simulink model "P4_RaspberryModel_with_DT"  (R2025b)
settings: Solver=daessc  StartTime=0.0  StopTime=Inf  FixedStep=0.01  RelTol=1e-3
PreLoadFcn:
  | % Kalman Filter testing
  | m=0.370;
  | l=0.075; %0.079793%determined by pendulum experiment %former values 0.032, 0.035;
  | lm=l*m; %lm=0.032*0.377
  | r=0.0405;
  | rm=r*m; %rm=0.0405*0.377
  | K=1;
  | 
  | tem=0.2 %initial guess
  | eta=2*lm+rm+(2*m*l^2/r);
  | 
  | A31=(lm+rm)/(tem*eta);
  | A32=9.81*lm/(r*eta);
  | A=[0 1 0 0; 0 -1/tem, 0, 0; 0, 0, 0, 1; 0 A31, A32, 0];
  | B=[0; 1/tem;0;-A31];
model workspace (MAT data in the model file):
  Amp = 1
undefined symbols (not defined in the file): anglerate, DiscIntNeverNeededParam, motor_left, motor_param, motor_right, PosEnc, VelEnc
libraries: simulink x19, raspberrypiCommlib x7, dspstat3 x6, slpidlib x3, sm_lib x3, raspberrypiNetworklib x2, svdutilitieslib x2, SigiLib x2, robotcorelib x1, mspfiltlib x1, nesl_utility x1
(part 2 of 2)

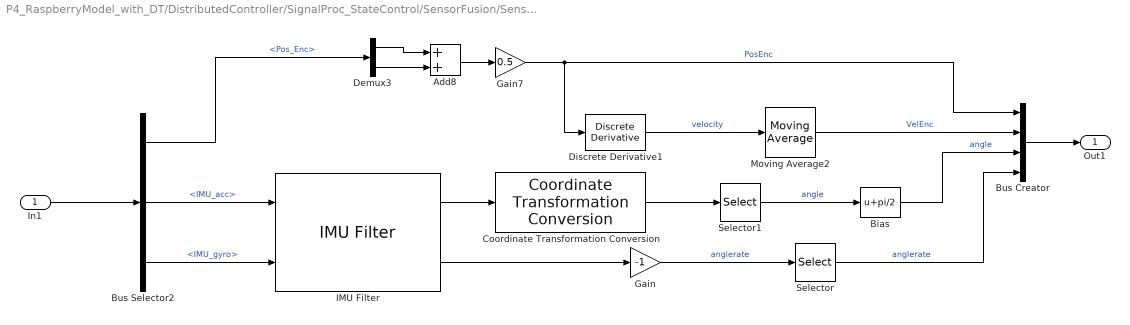
== system P4_RaspberryModel_with_DT/DistributedController/SignalProc_StateControl/SensorFusion/SensorFusion ==
  In1 : Inport
  Add8 : Sum
  Bias : Bias  Bias=pi/2  SaturateOnIntegerOverflow=off
  Bus Creator : BusCreator  Inputs=PosEnc,VelEnc,angle,anglerate  OutDataTypeStr=Bus: States
  Bus Selector2 : BusSelector  OutputSignals=Pos_Enc,IMU_acc,IMU_gyro
  Coordinate Transformation Conversion : robotcorelib/Coordinate Transformation Conversion  InputRepresentation=Rotation Matrix  InputEulerSequence=ZYX  ShowTrVecInputPort=on  OutputRepresentation=Euler Angles  OutputEulerSequence=XYZ  ShowTrVecOutputPort=on  SimulateUsing=Interpreted execution
      settings: LibrarySourceBlock=navlib/Utilities/Coordinate Transformation Conversion
  Demux3 : Demux  Outputs=2
  Discrete Derivative1 : simulink/Discrete/Discrete Derivative  gainval=1.0  ICPrevScaledInput=0.0  OutMin=[]  OutMax=[]  OutDataType=fixdt(1, 16)  OutScaling=2^-10  DoSatur=off
  Gain : Gain  Gain=-1
  Gain7 : Gain  Gain=0.5
  IMU Filter : mspfiltlib/IMU Filter  DispRefFrame=NED  OrientationFormat=Rotation matrix  DecimationFactor=1  InitialProcessNoise=imufilter.defaultProcessNoise  AccelerometerNoise=2.2693e-4  GyroscopeNoise=2.4065e-5  GyroscopeDriftNoise=3.0462e-13  LinearAccelerationNoise=0.0096236100000000012  LinearAccelerationDecayFactor=0.5  SimulateUsing=Interpreted execution
  Moving Average2 : dspstat3/Moving Average  Method=Sliding window  ForgettingFactorPort=off  SpecifyWindowLength=on  WindowLength=4  OverlapLength=3  AllowArbitraryInputLength=off  ForgettingFactor=0.9  SimulateUsing=Interpreted execution
  Selector : Selector  InputPortWidth=3  IndexOptions=Index vector (dialog)  Indices=[1]  OutputSizes=1
  Selector1 : Selector  InputPortWidth=3  IndexOptions=Index vector (dialog)  Indices=[1]  OutputSizes=1
  Out1 : Outport  OutDataTypeStr=Bus: States
  wires:
  Gain7/1 -> Bus Creator/1, Discrete Derivative1/1  "PosEnc"
  Demux3/2 -> Add8/2
  Discrete Derivative1/1 -> Moving Average2/1  "velocity"
  Bus Selector2/1 -> Demux3/1  "<Pos_Enc>"
  IMU Filter/1 -> Coordinate Transformation Conversion/1
  IMU Filter/2 -> Gain/1
  Bus Selector2/2 -> IMU Filter/1  "<IMU_acc>"
  Add8/1 -> Gain7/1
  Selector1/1 -> Bias/1  "angle"
  Bus Selector2/3 -> IMU Filter/2  "<IMU_gyro>"
  Demux3/1 -> Add8/1
  Coordinate Transformation Conversion/1 -> Selector1/1
  Selector/1 -> Bus Creator/4  "anglerate"
  Bus Creator/1 -> Out1/1
  In1/1 -> Bus Selector2/1
  Moving Average2/1 -> Bus Creator/2  "VelEnc"
  Bias/1 -> Bus Creator/3  "angle"
  Gain/1 -> Selector/1  "anglerate"

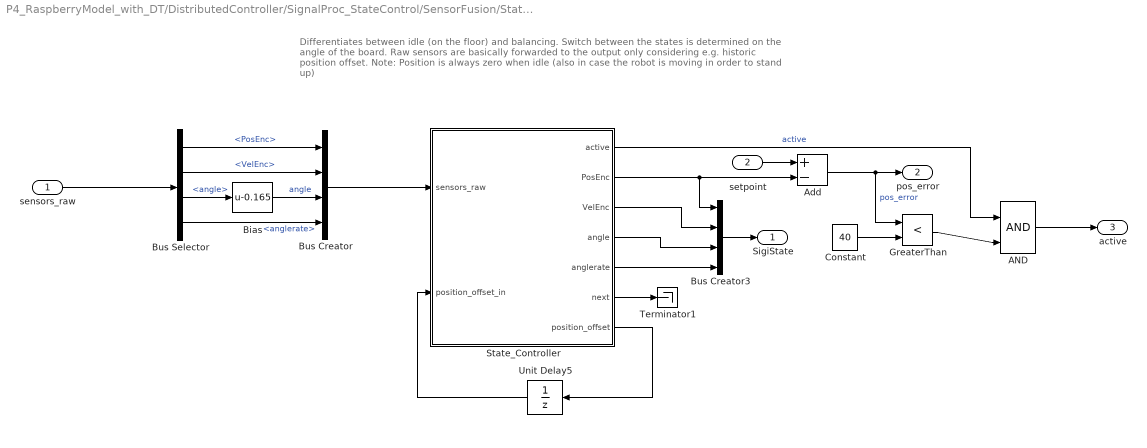
== system P4_RaspberryModel_with_DT/DistributedController/SignalProc_StateControl/SensorFusion/Statemachine ==
  note: Differentiates between idle (on the floor) and balancing.
      | Switch between the states is determined on the angle of the board.
      | Raw sensors are basically forwarded to the output only considering e.g. historic position offset.
      | Note: Position is always zero when idle (also in case the robot is moving in order to stand up)
  sensors_raw : Inport
  setpoint : Inport  Port=2
  AND : Logic  IconShape=distinctive  AllPortsSameDT=off  OutDataTypeStr=boolean
  Add : Sum  Inputs=+-
  Bias : Bias  Bias=-0.165  SaturateOnIntegerOverflow=off
  Bus Creator : BusCreator  Inputs=4  OutDataTypeStr=Bus: States
  Bus Creator3 : BusCreator  Inputs=PosEnc,VelEnc,angle,anglerate  OutDataTypeStr=Bus: States
  Bus Selector : BusSelector  OutputSignals=PosEnc,VelEnc,angle,anglerate
  Constant : Constant  Value=40  SampleTime=0.01
  GreaterThan : RelationalOperator  Operator=<  OutDataTypeStr=boolean  RndMeth=Simplest  InputSameDT=off
  State_Controller : Stateflow chart  TreatAsAtomicUnit=on
      settings: PortSchema="{\"entries\":[{\"content\":{\"sides\":[{\"content\":{\"connectorIds\":[\"In1\",\"In2\"]},\"type\":\"ConnectorPlacement.EquallySpacedRectSide\",\"uuid\":\"eb7aab9b-7b76-4287-a386-1fa94ac59388\"},{\"content\":{\"connectorIds\":[\"Out1\",\"Out4\",\"Out6\",\"Out5\",\"Out7\",\"Out2\",\"Out3\"],\"side\":\"RIGHT\"},\"type\":\"ConnectorPlacement.EquallySpacedRectSide\",\"uuid\":\"6af62896-360c-441a-abcb-d94064922169\"},{\"content\":{\"side\":\"TOP\"},\"type\":\"ConnectorPlacement.EquallySpacedRectSide\",\"uuid\":\"2e15ba59-a93a-45bf-98f2-d7da7205ed1e\"}]},\"type\":\"ConnectorPlacement.EquallySpacedConnector\",\"uuid\":\"1bfad314-89c0-4ae7-b541-c4839d2ff64d\"}],\"packageUris\":[\"http://schema.mathworks.com/mf0/Connector/R2020b\"],\"version\":\"1.0\"}"
  Terminator1 : Terminator
  Unit Delay5 : UnitDelay  SampleTime=-1  HasFrameUpgradeWarning=on
  SigiState : Outport  OutDataTypeStr=Bus: States
  pos_error : Outport  Port=2
  active : Outport  Port=3
  wires:
  Unit Delay5/1 -> State_Controller/2(position_offset_in)
  Bus Creator3/1 -> SigiState/1
  State_Controller/7(anglerate) -> Bus Creator3/4
  State_Controller/3(position_offset) -> Unit Delay5/1
  State_Controller/5(angle) -> Bus Creator3/3
  sensors_raw/1 -> Bus Selector/1
  State_Controller/4(PosEnc) -> Bus Creator3/1, Add/2
  State_Controller/1(active) -> AND/1  "active"
  State_Controller/2(next) -> Terminator1/1
  setpoint/1 -> Add/1
  Add/1 -> GreaterThan/1, pos_error/1  "pos_error"
  Constant/1 -> GreaterThan/2
  GreaterThan/1 -> AND/2
  AND/1 -> active/1
  State_Controller/6(VelEnc) -> Bus Creator3/2
  Bus Selector/3 -> Bias/1  "<angle>"
  Bias/1 -> Bus Creator/3  "angle"
  Bus Selector/4 -> Bus Creator/4  "<anglerate>"
  Bus Selector/2 -> Bus Creator/2  "<VelEnc>"
  Bus Selector/1 -> Bus Creator/1  "<PosEnc>"
  Bus Creator/1 -> State_Controller/1(sensors_raw)

== system P4_RaspberryModel_with_DT/SegwayDigitalTwin/RaspberryImplementation/LSM6DS33_IMU/Initialize Function ==
  note: Initiate the IMU - Setting sample rate and sensor range
  Constant : Constant  Value=64
  Constant2 : Constant  Value=64
  Data Type Conversion : DataTypeConversion  OutDataTypeStr=uint8  SaturateOnIntegerOverflow=off  RndMeth=Floor
  Data Type Conversion1 : DataTypeConversion  OutDataTypeStr=uint8  SaturateOnIntegerOverflow=off  RndMeth=Floor
  Event Listener : EventListener  DisableCoverage=on  EventName=reset
  I2C acc write : raspberrypiCommlib/I2C Controller Write  BoardProperty=Pi 3 Model B+  I2CModule=1  Mode=Master  SlaveAddress=107  SlaveByteOrder=BigEndian  Direction=Transmitter  RegisterAddressMode=on  RegisterAddress=16  SlaveDataType=uint8  DataLength=1  NoAck=off  RepeatedStart=off  OutputStatus=off
  I2C gyro write : raspberrypiCommlib/I2C Controller Write  BoardProperty=Pi 3 Model B+  I2CModule=1  Mode=Master  SlaveAddress=107  SlaveByteOrder=BigEndian  Direction=Transmitter  RegisterAddressMode=on  RegisterAddress=17  SlaveDataType=uint8  DataLength=1  NoAck=off  RepeatedStart=off  OutputStatus=off
  wires:
  Constant2/1 -> Data Type Conversion/1
  Data Type Conversion/1 -> I2C gyro write/1
  Data Type Conversion1/1 -> I2C acc write/1
  Constant/1 -> Data Type Conversion1/1

== system P4_RaspberryModel_with_DT/SegwayDigitalTwin/RaspberryImplementation/LSM6DS33_IMU/Terminate Function ==
  Constant : Constant  Value=0
  Constant2 : Constant  Value=0
  Data Type Conversion1 : DataTypeConversion  OutDataTypeStr=uint8  SaturateOnIntegerOverflow=off  RndMeth=Floor
  Data Type Conversion2 : DataTypeConversion  OutDataTypeStr=uint8  SaturateOnIntegerOverflow=off  RndMeth=Floor
  Event Listener : EventListener  DisableCoverage=on  EventType=Terminate  EventName=reset
  I2C Master Write : raspberrypiCommlib/I2C Controller Write  BoardProperty=Pi 3 Model B+  I2CModule=1  Mode=Master  SlaveAddress=107  SlaveByteOrder=BigEndian  Direction=Transmitter  RegisterAddressMode=on  RegisterAddress=17  SlaveDataType=uint8  DataLength=1  NoAck=off  RepeatedStart=off  OutputStatus=off
  I2C Master Write2 : raspberrypiCommlib/I2C Controller Write  BoardProperty=Pi 3 Model B+  I2CModule=1  Mode=Master  SlaveAddress=107  SlaveByteOrder=BigEndian  Direction=Transmitter  RegisterAddressMode=on  RegisterAddress=16  SlaveDataType=uint8  DataLength=1  NoAck=off  RepeatedStart=off  OutputStatus=off
  wires:
  Data Type Conversion1/1 -> I2C Master Write/1
  Constant/1 -> Data Type Conversion2/1
  Data Type Conversion2/1 -> I2C Master Write2/1
  Constant2/1 -> Data Type Conversion1/1

== system P4_RaspberryModel_with_DT/DistributedController/SignalProc_StateControl/ClassicalCalibration/SensorProcessing/BoardAngle ==
  note: This model only calculates the angle by comparing the relative magnitude of each component.
      | For the absolute acceleration one would need to use a calibration gain of 0.000488. (but sensor might drift...)
  x-sens : Inport  OutDataTypeStr=double
  z-sens : Inport  Port=2  OutDataTypeStr=double
  Atan2 : Trigonometry  Operator=atan2
  Gain1 : Gain  Commented=through  Gain=0.000488
  Gain2 : Gain  Commented=through  Gain=0.000488
  low pass filter : simulink/Discrete/Transfer Fcn First Order  PoleZ=0.95  ICPrevOutput=0.0  DoSatur=off
  Outport : Outport
  wires:
  x-sens/1 -> Gain2/1
  Gain1/1 -> Atan2/1
  Gain2/1 -> Atan2/2
  z-sens/1 -> Gain1/1
  Atan2/1 -> low pass filter/1  "board angle [rad]"
  low pass filter/1 -> Outport/1

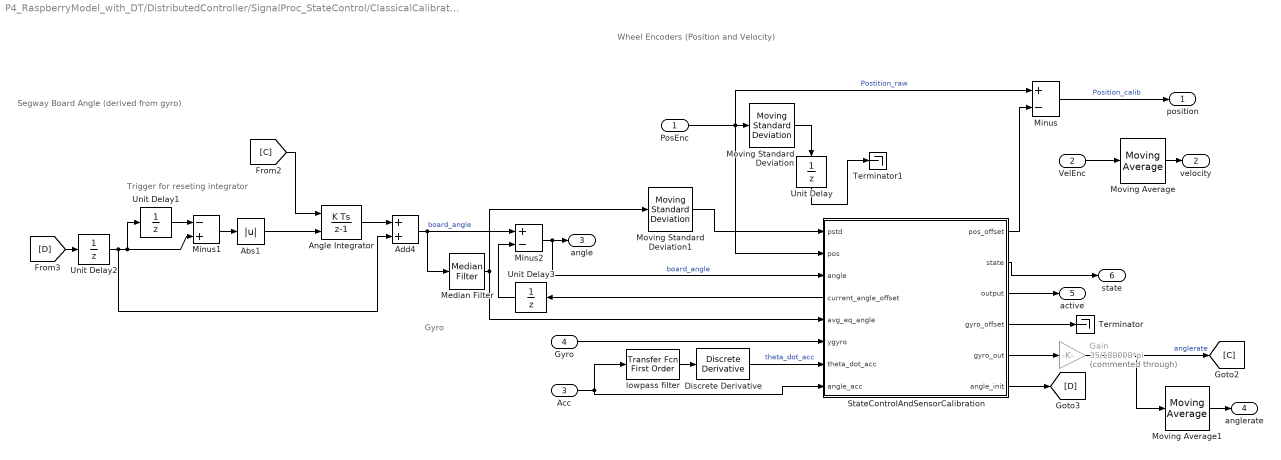
== system P4_RaspberryModel_with_DT/DistributedController/SignalProc_StateControl/ClassicalCalibration/Statemachine_Old/StateControl ==
  note: Segway Board Angle (derived from gyro)
  note: Wheel Encoders (Position and Velocity)
  note: Gyro
  note: Trigger for reseting integrator
  PosEnc : Inport
  VelEnc : Inport  Port=2
  Acc : Inport  Port=3
  Gyro : Inport  Port=4
  Abs1 : Abs  SaturateOnIntegerOverflow=off
  Add4 : Sum
  Angle Integrator : DiscreteIntegrator  gainval=1  ExternalReset=either  SampleTime=-1  ICPrevOutput=DiscIntNeverNeededParam  ICPrevScaledInput=DiscIntNeverNeededParam
  Discrete Derivative : simulink/Discrete/Discrete Derivative  gainval=1  ICPrevScaledInput=0.0  OutMin=[]  OutMax=[]  OutDataType=fixdt(1, 16)  OutScaling=2^-10  DoSatur=off
  Gain : Gain  Commented=through  Gain=35/180000*pi
  Median Filter : dspstat3/Median Filter  WindowLength=200  SimulateUsing=Interpreted execution
  Minus : Sum  Inputs=+-
  Minus1 : Sum  Inputs=-+
  Minus2 : Sum  Inputs=+-
  Moving Average : dspstat3/Moving Average  Method=Sliding window  ForgettingFactorPort=off  SpecifyWindowLength=on  WindowLength=4  OverlapLength=3  AllowArbitraryInputLength=off  ForgettingFactor=0.9  SimulateUsing=Code generation
  Moving Average1 : dspstat3/Moving Average  Method=Sliding window  ForgettingFactorPort=off  SpecifyWindowLength=on  WindowLength=4  OverlapLength=3  AllowArbitraryInputLength=off  ForgettingFactor=0.9  SimulateUsing=Code generation
  Moving Standard Deviation : dspstat3/Moving Standard Deviation  Method=Sliding window  ForgettingFactorPort=off  SpecifyWindowLength=on  WindowLength=200  OverlapLength=199  AllowArbitraryInputLength=off  ForgettingFactor=0.9  SimulateUsing=Code generation
  Moving Standard Deviation1 : dspstat3/Moving Standard Deviation  Method=Sliding window  ForgettingFactorPort=off  SpecifyWindowLength=on  WindowLength=200  OverlapLength=199  AllowArbitraryInputLength=off  ForgettingFactor=0.9  SimulateUsing=Code generation
  StateControlAndSensorCalibration : Stateflow chart  TreatAsAtomicUnit=on
      settings: PortSchema="{\"entries\":[{\"content\":{\"sides\":[{\"content\":{\"connectorIds\":[\"In6\",\"In1\",\"In2\",\"Out7\",\"In7\",\"In3\",\"In4\",\"In5\"]},\"type\":\"ConnectorPlacement.EquallySpacedRectSide\",\"uuid\":\"6d539330-cab8-492e-87fe-3819e6e7eb00\"},{\"content\":{\"connectorIds\":[\"Out1\",\"Out3\",\"Out2\",\"Out4\",\"Out5\",\"Out6\"],\"side\":\"RIGHT\"},\"type\":\"ConnectorPlacement.EquallySpacedRectSide\",\"uuid\":\"2301c18b-f8ee-47ce-b437-c31627e5a153\"},{\"content\":{\"side\":\"TOP\"},\"type\":\"ConnectorPlacement.EquallySpacedRectSide\",\"uuid\":\"43b5ca9c-e471-4dfa-b57b-f74bc9ed314e\"},{\"content\":{\"side\":\"BOTTOM\"},\"type\":\"ConnectorPlacement.EquallySpacedRectSide\",\"uuid\":\"e3357e76-5741-4d25-8fa4-a58b43fe78c4\"},{\"content\":{\"side\":\"HIDDEN\"},\"type\":\"ConnectorPlacement.EquallySpacedRectSide\",\"uuid\":\"7d6d1af1-4e73-4755-98b7-94e0e5692e13\"}]},\"type\":\"ConnectorPlacement.EquallySpacedConnector\",\"uuid\":\"634056c2-bd47-4d22-ad33-f1d4e41ccf21\"}],\"packageUris\":[\"http://schema.mathworks.com/mf0/Connector/R2020b\"],\"version\":\"1.0\"}"
  Terminator : Terminator
  Terminator1 : Terminator
  Unit Delay : UnitDelay  SampleTime=-1  HasFrameUpgradeWarning=on
  Unit Delay1 : UnitDelay  SampleTime=-1  HasFrameUpgradeWarning=on
  Unit Delay2 : UnitDelay  SampleTime=-1  HasFrameUpgradeWarning=on
  Unit Delay3 : UnitDelay  InitialCondition=0.19  SampleTime=-1  HasFrameUpgradeWarning=on
  lowpass filter : simulink/Discrete/Transfer Fcn First Order  PoleZ=0.95  ICPrevOutput=0.0  DoSatur=off
  position : Outport
  velocity : Outport  Port=2
  angle : Outport  Port=3
  anglerate : Outport  Port=4
  active : Outport  Port=5
  state : Outport  Port=6
  wires:
  Abs1/1 -> Angle Integrator/2
  PosEnc/1 -> Minus/1, StateControlAndSensorCalibration/1(pos), Moving Standard Deviation/1  "Postition_raw"
  Acc/1 -> StateControlAndSensorCalibration/5(angle_acc), lowpass filter/1
  Unit Delay1/1 -> Minus1/1
  Add4/1 -> Minus2/1, Median Filter/1  "board_angle"
  StateControlAndSensorCalibration/6(angle_init) -> [D]
  Discrete Derivative/1 -> StateControlAndSensorCalibration/4(theta_dot_acc)  "theta_dot_acc"
  Unit Delay2/1 -> Unit Delay1/1, Minus1/2, Add4/2
  lowpass filter/1 -> Discrete Derivative/1
  StateControlAndSensorCalibration/2(output) -> active/1
  StateControlAndSensorCalibration/1(pos_offset) -> Minus/2
  Angle Integrator/1 -> Add4/1
  StateControlAndSensorCalibration/5(gyro_out) -> Gain/1
  Minus/1 -> position/1  "Position_calib"
  Minus2/1 -> angle/1, StateControlAndSensorCalibration/2(angle)  "board_angle"
  Gyro/1 -> StateControlAndSensorCalibration/3(ygyro)
  [D] -> Unit Delay2/1
  Minus1/1 -> Abs1/1
  StateControlAndSensorCalibration/4(gyro_offset) -> Terminator/1
  Median Filter/1 -> StateControlAndSensorCalibration/7(avg_eq_angle), Moving Standard Deviation1/1
  Moving Standard Deviation/1 -> Unit Delay/1
  Unit Delay/1 -> Terminator1/1
  StateControlAndSensorCalibration/3(state) -> state/1
  StateControlAndSensorCalibration/7(current_angle_offset) -> Unit Delay3/1
  Unit Delay3/1 -> Minus2/2
  Moving Average1/1 -> anglerate/1
  [C] -> Angle Integrator/1
  Gain/1 -> [C], Moving Average1/1  "anglerate"
  Moving Standard Deviation1/1 -> StateControlAndSensorCalibration/6(pstd)
  Moving Average/1 -> velocity/1
  VelEnc/1 -> Moving Average/1

== system P4_RaspberryModel_with_DT/DistributedController/SignalProc_StateControl/SensorFusion/Statemachine/State_Controller/Balancing ==
  sensors_raw : Inport
  position_offset_in : Inport  Port=2
  Action Port : ActionPort
      settings: CopyFcn=Stateflow.SLINSF.SimulinkMan.removeBlockPreDeleteFcn  PreDeleteFcn=Stateflow.SLINSF.SimulinkMan.unsafePredeleteFcn
  Abs : Abs  SaturateOnIntegerOverflow=off
  Add : Sum  Inputs=-+
  Bus Selector1 : BusSelector  OutputSignals=PosEnc,VelEnc,angle,anglerate
  Compare To Constant : simulink/Logic and Bit Operations/Compare To Constant  relop=<=  const=pi/6  OutDataTypeStr=boolean
  Constant : Constant  SampleTime=0.01
  Switch : Switch  Criteria=u2 > Threshold  SaturateOnIntegerOverflow=off  InputSameDT=off
  active : Outport
  position_offset : Outport  Port=2
  PosEnc : Outport  Port=3
  VelEnc : Outport  Port=4
  angle : Outport  Port=5
  anglerate : Outport  Port=6
  wires:
  sensors_raw/1 -> Bus Selector1/1
  position_offset_in/1 -> Switch/1, Add/1
  Bus Selector1/3 -> angle/1, Abs/1  "<angle>"
  Constant/1 -> active/1
  Compare To Constant/1 -> Switch/2
  Abs/1 -> Compare To Constant/1
  Bus Selector1/1 -> Add/2  "<PosEnc>"
  Bus Selector1/2 -> VelEnc/1  "<VelEnc>"
  Add/1 -> Switch/3, PosEnc/1  "PosEnc"
  Bus Selector1/4 -> anglerate/1  "<anglerate>"
  Switch/1 -> position_offset/1

== system P4_RaspberryModel_with_DT/DistributedController/SignalProc_StateControl/SensorFusion/Statemachine/State_Controller/Out ==
  sensors_raw : Inport
  Action Port : ActionPort
      settings: CopyFcn=Stateflow.SLINSF.SimulinkMan.removeBlockPreDeleteFcn  PreDeleteFcn=Stateflow.SLINSF.SimulinkMan.unsafePredeleteFcn
  Bus Selector1 : BusSelector  OutputSignals=PosEnc,VelEnc,angle,anglerate
  Constant : Constant  Value=0  SampleTime=0.01
  Constant3 : Constant  Value=0  SampleTime=0.01
  active : Outport
  PosEnc : Outport  Port=2
  VelEnc : Outport  Port=3
  angle : Outport  Port=4
  anglerate : Outport  Port=5
  position_offset : Outport  Port=6
  wires:
  sensors_raw/1 -> Bus Selector1/1
  Bus Selector1/1 -> position_offset/1  "<PosEnc>"
  Bus Selector1/3 -> angle/1  "<angle>"
  Bus Selector1/4 -> anglerate/1  "<anglerate>"
  Constant3/1 -> active/1
  Bus Selector1/2 -> VelEnc/1  "<VelEnc>"
  Constant/1 -> PosEnc/1

== matlab function P4_RaspberryModel_with_DT/SegwayDigitalTwin/RaspberryImplementation/AlignSensorAxes ==
  data: u1 input; y output; u2 input; u3 input
function y = fcn(u1,u2,u3)

y = [-u2 u1 u3];

== matlab function P4_RaspberryModel_with_DT/SegwayDigitalTwin/RaspberryImplementation/AlignSensorAxes1 ==
  data: u1 input; y output; u2 input; u3 input
function y = fcn(u1,u2,u3)

y = [u2 u1 u3];

== stateflow chart P4_RaspberryModel_with_DT/DistributedController/SignalProc_StateControl/ClassicalCalibration/Statemachine_Old/StateControl/StateControlAndSensorCalibration ==
  state GyroCalibration
    %stable orientation -> good to calibrate the gyro
    entry:
    state=1.1;
    t=0;
    gyro=0;
    during:
    t=t+1;
    gyro=gyro+ygyro;
    exit: %define the angle measurement output
    gyro_offset=gyro/t;
    pos_offset=pos;
    angle_init=angle_acc;
  state Balancing
    entry:
    output=1;
    state=3;
    t=0
    during:
    t=t+1
    gyro_out=ygyro-gyro_offset
  state BalDriftComp
    during:
    state=4;
    current_angle_offset=avg_eq_angle;
    gyro_out=ygyro-gyro_offset;
  state Wait
    entry:
    gyro_out=0;
    output=0;
    state=1;
    angle_init=0;
    current_angle_offset=0.19;
    %check if there is no change in angle
  state Idle
    entry:
    state=2;
    output=0;
    during:
    gyro_out=ygyro-gyro_offset
  (default) -> Wait
  Balancing -> BalDriftComp [order 2] : [t>=200 && pstd<=0.005]
  Wait -> GyroCalibration : [abs(theta_dot_acc)<=0.008]
  Idle -> Balancing : [abs(angle)<=pi/4]
  GyroCalibration -> Idle [order 2] : [t>=100]
  BalDriftComp -> Balancing [order 2] : [pstd>0.005]
  GyroCalibration -> Wait [order 1] : [abs(theta_dot_acc)>0.01]
  BalDriftComp -> Wait [order 1] : [abs(angle)>pi/5]
  Balancing -> Wait [order 1] : [abs(angle)>0.8]
  data: pos_offset output; pos input; t local; angle input; ygyro input; gyro local; theta_dot_acc input; output output; angle_acc input; state output; gyro_offset output; gyro_out output; angle_init output; pstd input; current_angle_offset output; avg_eq_angle input

== stateflow chart P4_RaspberryModel_with_DT/DistributedController/SignalProc_StateControl/SensorFusion/Statemachine/State_Controller ==
  state Out
  state Balancing
  (default) -> Out
  Out -> Balancing : [abs(angle)<pi/6]
  Balancing -> Out : [abs(angle)>=pi/6]
  data: sf_internal_action_state_placeholder_data local double size=1 =0; sf_internal_action_state_placeholder_data local double size=1 =0; active output size=1; next output double size=1; sensors_raw input Bus: States; position_offset output; PosEnc output; angle output =pi; VelEnc output; anglerate output; position_offset_in input
